simulink model "QAM16_constellation_IQ"  (R2021a)
settings: Solver=VariableStepDiscrete  StartTime=0.0  StopTime=1000/fs  RelTol=1e-3  EnableMultiTasking=on
PreLoadFcn:
  | %%%%%%%%%%%%%%%%%%%%%%%%%%%%%%%%%%%%%%%%%%%%%%%%%%%%%%%%%%%%%%%%%%%%%%%%%%%
  | % check to see if Simulink library folder is missing from the MATLAB path %
  | %%%%%%%%%%%%%%%%%%%%%%%%%%%%%%%%%%%%%%%%%%%%%%%%%%%%%%%%%%%%%%%%%%%%%%%%%%%
  | if isempty(strfind(path, 'rtlsdr_book_library'))
  | 
  |     % create error window
  |     fig_error = figure(...
  |         'Name', 'Error: RTL-SDR Book Library',...
  |         'Toolbar','none',...
  |         'MenuBar','none',...
  |         'NumberTitle','off',...
  |         'Resize','off',...
  |         'WindowStyle','modal');
  |     fig_error.Position(3) = 600;
  |     fig_error.Position(4) = 150;
  |     fig_axes = axes(...
  |         'Parent',fig_error,...
  |         'Position',[0,0,1,1],...
  |         'visible','off');
  |     % error message
  |     t_title = text(.05,.8,...
  |         'MISSING DIRECTORIES',...
  |         'FontSize',11.5);
  |     t_body = text(.075,.6,...
  |         [{'Simulink cannot find the  \it{<root>}\rm / \it{rtlsdr\_book\_library}\rm  folder in the \it{MATLAB Path}\rm.'},...
  |         {'Please set the MATLAB path following the instructions given in Exercise 2.4.'}],...
  |         'FontSize',10.5);
  |     % buttons
  |     btn_path = uicontrol(...
  |         'Parent',fig_error,...
  |         'String','Set Path Now',...
  |         'FontSize',10,...
  |         'Callback', 'pathtool; close(fig_error);',...
  |         'Position', [fig_error.Position(3)/2-210, 30, 200, 30]);
  |     btn_abort = uicontrol(...
  |         'Parent',fig_error,...
  |         'String','No thanks',...
  |         'FontSize',10,...
  |         'Callback', 'close(fig_error); abort=1;',...
  |         'Position', [fig_error.Position(3)/2+10, 30, 200, 30]);
  | 
  |     % pause to allow user to interact with error box
  |     uiwait(fig_error);
  | 
  |     % abort simulation
  |     try
  |         if abort==1
  |             set_param(gcs, 'SimulationCommand', 'stop');
  |         end
  |     end
  | 
  |     % if user has set path, allow diagram to be updated
  |     if ~exist('abort','var')
  |         % create error window
  |         fig_update = figure(...
  |             'Name', 'Update Diagram',...
  |             'Toolbar','none',...
  |             'MenuBar','none',...
  |             'NumberTitle','off',...
  |             'Resize','off');
  |         fig_update.Position(3) = 400;
  |         fig_update.Position(4) = 120;
  |         fig_axes = axes(...
  |             'Parent',fig_update,...
  |             'Position',[0,0,1,1],...
  |             'visible','off');
  |         % instruction message
  |         t_body = text(.075,.7,...
  |             'Once you have set the path, update the block diagram',...
  |             'FontSize',10.5);
  |         % button
  |         btn_update = uicontrol(...
  |             'Parent',fig_update,...
  |             'String','Update Block Diagram',...
  |             'FontSize',10,...
  |             'Callback', 'set_param(gcs,''SimulationCommand'',''update''); close(gcf)',...
  |             'Position', [fig_update.Position(3)/2-100, 30, 200, 30]);
  |     end
  | 
  |     % clear error components
  |     clear('fig_error','fig_update','fig_axes','t_title','t_body','btn_path','btn_abort','btn_update','abort');
  | 
  | end
  | %%%%%%%%%%%%%%%%%%%%%%%%%%%%%%%%%%%%%%%%%%%%%%%%%%%%%%%%%%%%%%%%%%%%%%%%%%%
  | 
  | MHz = 100;
  | fs = MHz * 1e6;
  | 
  | % setup reference constellation points
  | qam16_points = [-1-i, -1-i/3, -1+i/3, -1+i;
  |                          -1/3-i, -1/3-i/3, -1/3+i/3, -1/3+i;
  |                          1/3-i, 1/3-i/3, 1/3+i/3, 1/3+i;
  |                          1-i, 1-i/3, 1+i/3, 1+i];
libraries: commchan3 x2, commdigbbndam3 x2, commrandsrc3 x1, rtlsdr_book_library x1
CloseFcn:
  | closefcn_model;
Description:
  | Software, Simulation Examples and Design Exercises Licence Agreement
  | 
  | This license agreement refers to the simulation examples, design exercises and files,
  | and associated software MATLAB and Simulink resources that accompany the book:
  | 
  |      Title: Software Defined Radio using MATLAB & Simulink and the RTL-SDR
  |      Published by Strathclyde Academic Media, 2015
  |      Authored by Robert W. Stewart, Kenneth W. Barlee, Dale S.W. Atkinson,
  |      and Louise H. Crockett
  | 
  | and made available as a download from, www.desktopSDR.com or variously acquired
  | by other means such as via USB storage, cloud storage, disk or any other electronic
  | or optical or magnetic storage mechanism. These files and associated software may
  | be used subject to the terms of agreement of the conditions below:
  | 
  |     Copyright © 2015 Robert W. Stewart, Kenneth W. Barlee, Dale S.W. Atkinson,
  |     and Louise H. Crockett
  |     All rights reserved.
  | 
  | Redistribution and use in source and binary forms, with or without modification, are
  | permitted provided that the following conditions are met:
  | 
  |    1.  Redistributions of source code must retain the above copyright notice, this list of
  |         conditions and the following disclaimer.
  | 
  |    2.  Redistributions in binary form must reproduce the above copyright notice, this
  |         list of conditions and the following disclaimer in the documentation and/or other
  |         materials provided with the distribution.
  | 
  |    3.  Neither the name of the copyright holder nor the names of its contributors may
  |         be used to endorse or promote products derived from this software without
  |         specific prior written permission.
  | 
  |    4.  In all cases, the software is, and all modifications and derivatives of the
  |         software shall be, licensed to you solely for use in conjunction with The
  |         MathWorks, Inc. products and service offerings.
  | 
  | THIS SOFTWARE IS PROVIDED BY THE COPYRIGHT HOLDERS AND CONTRIBUTORS
  | "AS IS" AND ANY EXPRESS OR IMPLIED WARRANTIES, INCLUDING, BUT NOT LIMITED
  | TO, THE IMPLIED WARRANTIES OF MERCHANTABILITY AND FITNESS FOR A
  | PARTICULAR PURPOSE ARE DISCLAIMED. IN NO EVENT SHALL THE COPYRIGHT
  | HOLDER OR CONTRIBUTORS BE LIABLE FOR ANY DIRECT, INDIRECT, INCIDENTAL,
  | SPECIAL, EXEMPLARY, OR CONSEQUENTIAL DAMAGES (INCLUDING, BUT NOT
  | LIMITED TO, PROCUREMENT OF SUBSTITUTE GOODS OR SERVICES; LOSS OF USE,
  | DATA, OR PROFITS; OR BUSINESS INTERRUPTION) HOWEVER CAUSED AND ON ANY
  | THEORY OF LIABILITY, WHETHER IN CONTRACT, STRICT LIABILITY, OR TORT
  | (INCLUDING NEGLIGENCE OR OTHERWISE) ARISING IN ANY WAY OUT OF THE USE
  | OF THIS SOFTWARE, EVEN IF ADVISED OF THE POSSIBILITY OF SUCH DAMAGE.
  | 
  | 
  | Audio Tracks used in Simulations Examples and Design Exercises
  | 
  | The music and vocal files used within the Examples files and software within the book
  | were variously written, arranged, performed, recorded and produced by Garrey Rice,
  | Adam Struth, Jamie Struth, Iain Thistlethwaite and also Marshall Craigmyle who
  | collectively, and individually where appropriate, assert and retain all of their copyright,
  | performance and artistic rights. Permission to use and reproduce this music is
  | granted for all purposes associated with MATLAB and Simulink software and the
  | simulation examples and design exercises files that accompany this book. Requests to
  | use the music for any other purpose should be directed to: info@desktopSDR.com.
  | For information on music track names, full credits, and links to the musicians please
  | refer to www.desktopSDR.com/more/audio.
settings Model: Creator=desktopSDR Team  LastModifiedBy=Alex
settings SolverCC: AlgebraicLoopSolver=TrustRegion
settings DataIOCC: SaveFormat=Array  SaveOutput=off  SignalLogging=off  SaveTime=off  ReturnWorkspaceOutputs=off
settings OptimizationCC: LifeSpan=inf
settings DebuggingCC: UnderspecifiedInitializationDetection=Classic  MergeDetectMultiDrivingBlocksExec=none  SolverPrmCheckMsg=warning  SFUnexpectedBacktrackingDiag=warning  SFNoUnconditionalDefaultTransitionDiag=warning  SFExecutionAtInitializationDiag=none  SFMachineParentedDataDiag=warning  ArithmeticOperatorsInVariantConditions=warning
settings HardwareCC: ProdBitPerPointer=32  ProdBitPerSizeT=32  ProdBitPerPtrDiffT=32  ProdLargestAtomicFloat=None  ProdIntDivRoundTo=Undefined  ProdEndianess=Unspecified  ProdWordSize=32  ProdHWDeviceType=32-bit Generic
settings ModelReferenceCC: PropagateSignalLabelsOutOfModel=off
settings SFSimCC: SimUseLocalCustomCode=off  CustomCodeUndefinedFunction=UseInterfaceOnly
settings RTWCC: RTWUseLocalCustomCode=off
settings CodeAppCC: StateflowObjectComments=on
settings GRTTargetCC: TargetLangStandard=C89/C90 (ANSI)
settings ConfigComp: CovMetricSettings=dw  CovSaveCumulativeToWorkspaceVar=on  CovSaveSingleToWorkspaceVar=on  CovExternalEMLEnable=off  CovSFcnEnable=off

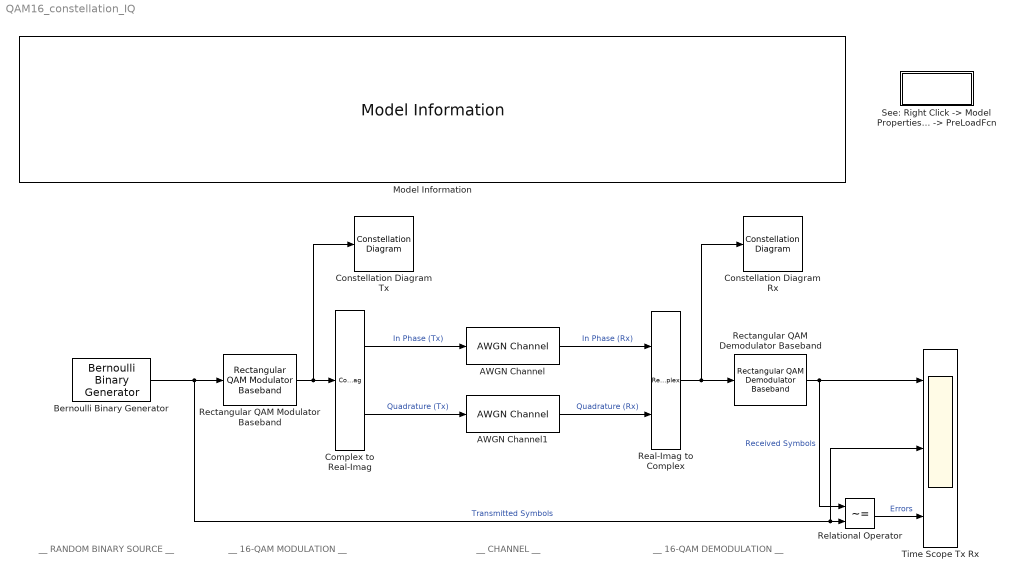
== system QAM16_constellation_IQ ==
  note: __ RANDOM BINARY SOURCE __
  note: __ 16-QAM MODULATION __
  note: __ 16-QAM DEMODULATION __
  note: __ CHANNEL __
  AWGN Channel : commchan3/AWGN Channel  InputProcessing=Columns as channels (frame based)  seed=673  noiseMode="Signal to noise ratio  (Eb/No)"  EbNodB=20  EsNodB=10  SNRdB=10  bitsPerSym=2  Ps=1  Tsym=4/fs  variance=1
  AWGN Channel1 : commchan3/AWGN Channel  InputProcessing=Columns as channels (frame based)  seed=67  noiseMode="Signal to noise ratio  (Eb/No)"  EbNodB=20  EsNodB=10  SNRdB=10  bitsPerSym=2  Ps=1  Tsym=4/fs  variance=1
  Bernoulli Binary Generator : commrandsrc3/Bernoulli Binary Generator  ProbabilityOfZero=0.5  SeedSource=Parameter  Seed=61  SampleTime=1/fs  SamplesPerFrame=4  OutputDataType=boolean  SimulateUsing=Interpreted execution
  Complex to Real-Imag : ComplexToRealImag
  Constellation Diagram Rx : ConstellationDiagram
  Constellation Diagram Tx : ConstellationDiagram
  Model Information : rtlsdr_book_library/Additional Tools/Model Information/Model Information
      settings: SourceProductName=RTL-SDR Book Library
  Real-Imag to Complex : RealImagToComplex
  Rectangular QAM Demodulator Baseband : commdigbbndam3/Rectangular QAM Demodulator Baseband  M=16  OutType=Bit  DecType=Hard decision  VarSource=Dialog  Variance=1  Dec=Gray  Mapping=[0:15]  PowType=Min. distance between symbols  MinDist=2/3  AvgPow=1  PeakPow=1  Ph=0  outDtype1=Inherit via internal rule  outDtype2=Inherit via internal rule  derotateFactorWordLen=16  derotateFactorDataTypeStr=Inherit: Same word length as input  derotateFactorLastDataTypeStr=Inherit: Same word length as input  denormFactorWordLen=16  denormFactorDataTypeStr=Inherit: Same word length as input  denormFactorLastDataTypeStr=Inherit: Same word length as input  prodOutWordLen=32  prodOutOverflowMode=Wrap  prodOutRoundingMode=Floor  prodOutOvFlMode=off  prodOutOvFlModeLastStrValue=off  sumWordLen=32
  Rectangular QAM Modulator Baseband : commdigbbndam3/Rectangular QAM Modulator Baseband  M=16  InType=Bit  Enc=Gray  Mapping=[0:15]  PowType=Min. distance between symbols  MinDist=2/3  AvgPow=1  PeakPow=1  Ph=0  outDtype=double  outWordLen=16  outUDDataType=sfix(16)  outFracLenMode=User-defined  outFracLen=14  outDataTypeStr=double  outLastDataTypeStr=double
  Relational Operator : RelationalOperator  Operator=~=  OutDataTypeStr=boolean  RndMeth=Nearest
  "See: Right Click -> Model Properties -> Callbacks -> PreLoadFcn " : Subsystem
      mask Display:
      | MHz = evalin('base', 'MHz');
      | fprintf(['fs = ',num2str(MHz),' MHz']);
  Time Scope Tx Rx : Scope  NumInputPorts=3
  wires:
  Bernoulli Binary Generator/1 -> Time Scope Tx Rx/2, Relational Operator/2, Rectangular QAM Modulator Baseband/1  "Transmitted Symbols"
  Rectangular QAM Demodulator Baseband/1 -> Time Scope Tx Rx/1, Relational Operator/1  "Received Symbols"
  Relational Operator/1 -> Time Scope Tx Rx/3  "Errors"
  Rectangular QAM Modulator Baseband/1 -> Constellation Diagram Tx/1, Complex to Real-Imag/1
  Real-Imag to Complex/1 -> Constellation Diagram Rx/1, Rectangular QAM Demodulator Baseband/1
  Complex to Real-Imag/1 -> AWGN Channel/1  "In Phase (Tx)"
  AWGN Channel/1 -> Real-Imag to Complex/1  "In Phase (Rx)"
  Complex to Real-Imag/2 -> AWGN Channel1/1  "Quadrature (Tx)"
  AWGN Channel1/1 -> Real-Imag to Complex/2  "Quadrature (Rx)"

== system QAM16_constellation_IQ/See: Right Click -> Model Properties -> Callbacks -> PreLoadFcn  ==
